simulink model "NonLinearResistor"  (R2018b)
settings: Solver=FixedStepDiscrete  StartTime=0.0  StopTime=10  FixedStep=Ts  RelTol=1e-3
PreLoadFcn:
  | setMatlabPaths
  | Ts = 1e-3
libraries: Simple_lib x3
settings Model: PauseTimes=1  NumberOfSteps=100  Creator=billw  LastModifiedBy=billw
settings DataIOCC: SignalLogging=off  DSMLogging=off

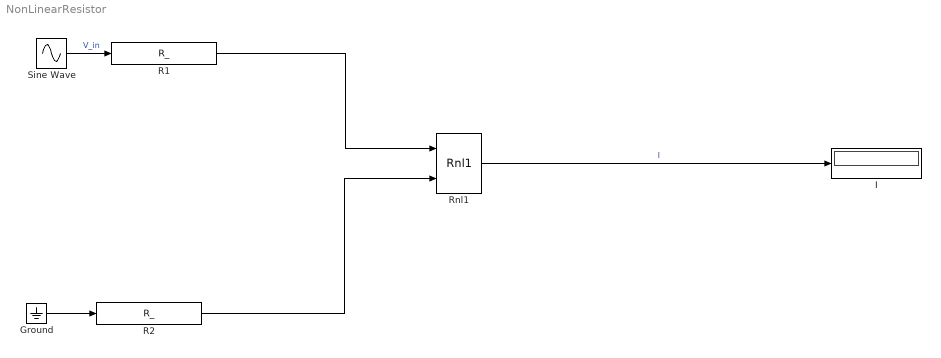
== system NonLinearResistor ==
  Ground : Ground
  I : Display
  R1 : Simple_lib/Electronics/R_  Exponent=0  R=1
      settings: AttributesFormatString=%<R> Ohm
  R2 : Simple_lib/Electronics/R_  Exponent=0  R=1
      settings: AttributesFormatString=%<R> Ohm
  Rnl1 : Simple_lib/Electronics/Rnl1  I_S=1e-12  n=2  T_def=300
  Sine Wave : Sin  Amplitude=2  Frequency=10*pi  SampleTime=0
  wires:
  Sine Wave/1 -> R1/1  "V_in"
  Ground/1 -> R2/1
  Rnl1/1 -> I/1  "I"
  R2/1 -> Rnl1/2
  R1/1 -> Rnl1/1
